simulink model "Motor_Diesel"  (R2017a)
settings: Solver=VariableStepAuto  StartTime=0.0  StopTime=1000  RelTol=1e-3  EnableMultiTasking=on
undefined symbols (not defined in the file): J, K1, K2, K3, P, Tao1, Tao2
settings Model: Creator=dmartinez  LastModifiedBy=erich
settings OptimizationCC: LifeSpan=inf
settings DebuggingCC: SFUnexpectedBacktrackingDiag=warning  SFNoUnconditionalDefaultTransitionDiag=warning  SFExecutionAtInitializationDiag=none
settings GRTTargetCC: TargetLangStandard=C89/C90 (ANSI)  GeneratePreprocessorConditionals=Disable all
settings ConfigComp: CovMetricSettings=dw  CovHtmlReporting=on  CovSaveCumulativeToWorkspaceVar=on  CovSaveSingleToWorkspaceVar=on  CovExternalEMLEnable=off

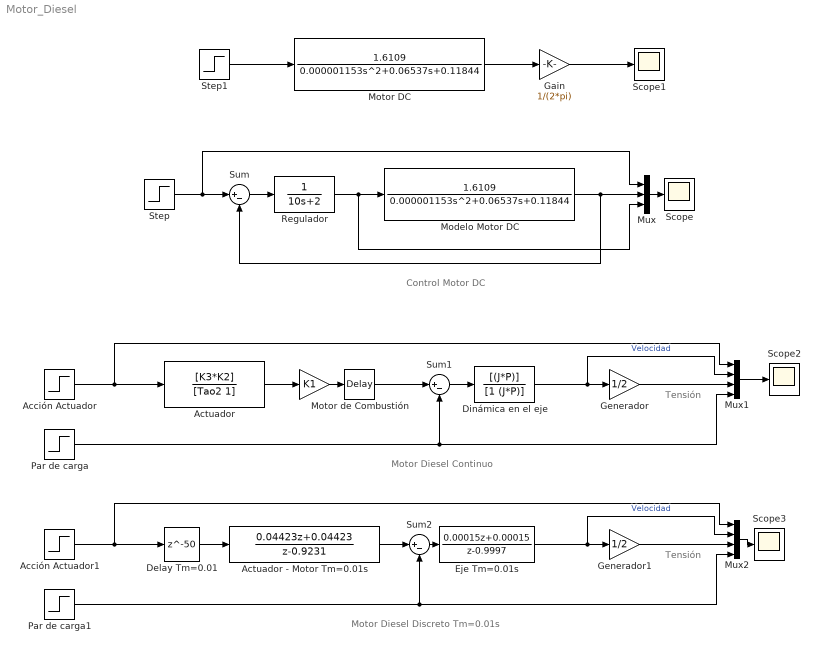
== system Motor_Diesel ==
  note: Motor Diesel Continuo
  note: Control Motor DC
  note: Tensión
  note: Motor Diesel Discreto Tm=0.01s
  note: Tensión
  " " : Gain  Gain=K1
  " Generador" : Gain  Gain=1/2
  " Generador1" : Gain  Gain=1/2
  Acción Actuador : Step  Time=0  SampleTime=0
  Acción Actuador1 : Step  Time=0  SampleTime=0
  Actuador : TransferFcn  Numerator=[K3*K2]  Denominator=[Tao2 1]
  Actuador - Motor Tm=0.01s : DiscreteTransferFcn  Numerator=[0.04423 0.04423]  Denominator=[1 -0.9231]  SampleTime=0.01
  Delay Tm=0.01 : Delay  DelayLength=50  SampleTime=0.01
  Dinámica en el eje : TransferFcn  Numerator=[(J*P)]  Denominator=[1 (J*P)]
  Eje Tm=0.01s : DiscreteTransferFcn  Numerator=[0.00015 0.00015]  Denominator=[1 -0.9997]  SampleTime=0.01
  Gain : Gain  Gain=1/(2*pi)
  Modelo Motor DC : TransferFcn  Numerator=[1.6109]  Denominator=[0.000001153 0.06537 0.11844]
  Motor DC : TransferFcn  Numerator=[1.6109]  Denominator=[0.000001153 0.06537 0.11844]
  Motor de Combustión : TransportDelay  DelayTime=Tao1
  Mux : Mux  Inputs=3
  Mux1 : Mux
  Mux2 : Mux
  Par de carga : Step  Time=300  Before=0.1  SampleTime=0
  Par de carga1 : Step  Time=300  Before=0.1  SampleTime=0
  Regulador : TransferFcn  Denominator=[10 2]
  Scope{,1..3} (4 alike) : Scope
  Step : Step  SampleTime=0
  Step1 : Step  Time=0  SampleTime=0
  Sum : Sum  Inputs=|+-
  Sum1 : Sum  Inputs=|+-
  Sum2 : Sum  Inputs=|+-
  wires:
  Sum/1 -> Regulador/1
  Step/1 -> Mux/1, Sum/1
  Mux/1 -> Scope/1
  Step1/1 -> Motor DC/1
  Regulador/1 -> Mux/3, Modelo Motor DC/1
  Motor DC/1 -> Gain/1
  Gain/1 -> Scope1/1
  Modelo Motor DC/1 -> Sum/2, Mux/2
  Mux1/1 -> Scope2/1
  Actuador/1 -> " "/1
  " "/1 -> Motor de Combustión/1
  Motor de Combustión/1 -> Sum1/1
  Sum1/1 -> Dinámica en el eje/1
  Dinámica en el eje/1 -> Mux1/2, " Generador"/1  "Velocidad"
  Acción Actuador/1 -> Mux1/1, Actuador/1
  " Generador"/1 -> Mux1/3
  Par de carga/1 -> Mux1/4, Sum1/2
  Mux2/1 -> Scope3/1
  Sum2/1 -> Eje Tm=0.01s/1
  Eje Tm=0.01s/1 -> Mux2/2, " Generador1"/1  "Velocidad"
  Acción Actuador1/1 -> Delay Tm=0.01/1, Mux2/1
  " Generador1"/1 -> Mux2/3
  Par de carga1/1 -> Mux2/4, Sum2/2
  Delay Tm=0.01/1 -> Actuador - Motor Tm=0.01s/1
  Actuador - Motor Tm=0.01s/1 -> Sum2/1
